simulink model "d2kontur_d2"  (R2014b)
settings: Solver=ode3  SolverMode=SingleTasking  StartTime=0.0  StopTime=10.0  RelTol=1e-3
PreLoadFcn:
  | waijung.modelPreload; % Required for working with Waijung Blockset. Do not remove.
undefined symbols (not defined in the file): FiO2, HCLK, HSEOSC, Link, LQFP100, ST, STM32F407VE
libraries: simulink_extras x8, stm32f4_io_lib x2, stm32f4_adc_lib x1, stm32f4_device_config_lib x1
(part 1 of 2)
CloseFcn:
  | waijung.modelClose; % Required for working with Waijung Blockset. Do not remove.
settings Model: Creator=Алексей  LastModifiedBy=Alex
settings OptimizationCC: OptimizeModelRefInitCode=on  LifeSpan=1
settings HardwareCC: ProdEndianess=LittleEndian  ProdHWDeviceType=ARM Compatible->Cortex - M4  TargetEndianess=LittleEndian  TargetHWDeviceType=ARM Compatible->Cortex - M4
settings RTWCC: SystemTargetFile=stm32f4.tlc  GenerateMakefile=off  TemplateMakefile=ert_default_tmf  Description=STM32F4 Target  ProcessScript=stm32f4_make_rtw_hook
settings CodeAppCC: IgnoreCustomStorageClasses=off
settings STFCustomTargetCC: ModelReferenceCompliant=off  CombineOutputUpdateFcns=on  ERTCustomFileBanners=on  SupportContinuousTime=off  SupportNonInlinedSFcns=off  MATLABClassNameForMDSCustomization=Simulink.SoftwareTarget.ERTCustomization  GRTInterface=off  SystemTargetFile=stm32f4.tlc
settings ERTTargetCC: ModelReferenceCompliant=off  ParMdlRefBuildCompliant=off  CompOptLevelCompliant=off  ConcurrentExecutionCompliant=off  ERTFirstTimeCompliant=off  ModelStepFunctionPrototypeControlCompliant=off  CPPClassGenCompliant=off  InlinedParameterPlacement=NonHierarchical  ERTSrcFileBannerTemplate=stm32f4_code_template.cgt  ERTHdrFileBannerTemplate=stm32f4_code_template.cgt  ERTDataSrcFileTemplate=stm32f4_code_template.cgt  ERTDataHdrFileTemplate=stm32f4_code_template.cgt  ERTCustomFileTemplate=stm32f4_file_process.tlc

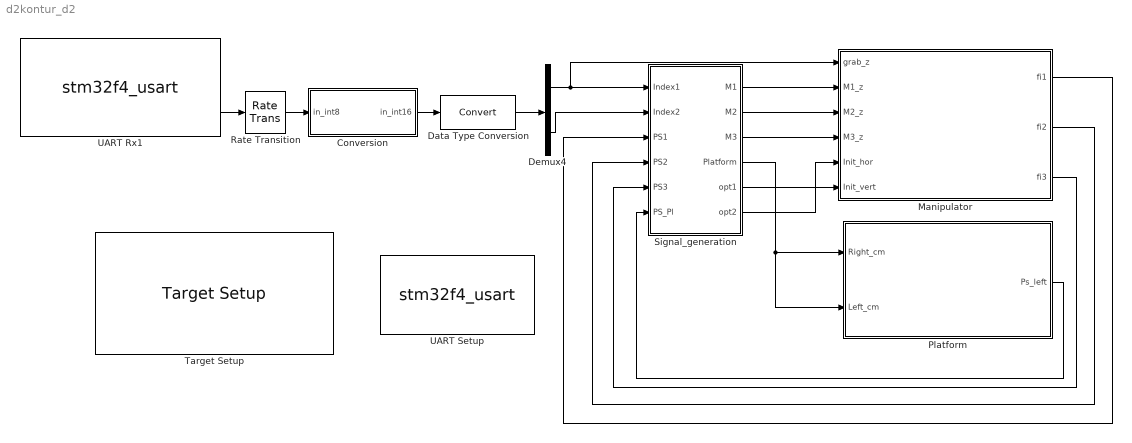
== system d2kontur_d2 ==
  Conversion : Subsystem
  Data Type Conversion : DataTypeConversion
  Demux4 : Demux  Outputs=2
  Manipulator : Subsystem
      mask Display:
      | port_label('input',1,'grab')
      | port_label('input',2,'M1')
      | port_label('input',3,'M2')
      | port_label('input',4,'M3')
      | port_label('input',5,'Init_h')
      | port_label('input',6,'Init_v')
      | port_label('output',1,'fi1')
      | port_label('output',2,'fi2')
      | port_label('output',3,'fi3')
  Platform : Subsystem
  Rate Transition : RateTransition  OutPortSampleTime=0.001
  Signal_generation : Subsystem
  Target Setup : stm32f4_device_config_lib/Target Setup  Priority=100  compiler=GNU ARM  previous_compiler=GNU ARM  mcu=STM32F407VE (LQFP100)  mcustr=STM32F407VE  clockconfig=FiO2 (HSEOSC-8MHz/HCLK-168MHz)  system_stm32f4xx_c_path=C:\waijung15_04a\targets\stm32f4_target\stm32f4\utils\STM32F4xx_AN3988_V1.0.1\stm32f4_default\hseosc8mhz  showmemoryconfiguration=off  stacksize=0x2000  heapsize=0x2000  enableautocompiledownload=on  fullchiperase=off  programmerinterface=ST-Link  editctrlstr=on  compilercontrolstr=$(patsubst %, -I%, .) -mcpu=cortex-m4 -mthumb -mthumb-interwork -mfloat-abi=hard -mfpu=fpv4-sp-d16 -ffast-math -Wall -Wextra -Ofast  assemblercontrolstr=$(patsubst %, -I%, .) -mcpu=cortex-m4 -mthumb -mthumb-interwork -mfloat-abi=hard -mfpu=fpv4-sp-d16 -ffast-math -Wall -Wextra -Ofast -Wa,-amhls=$(<:.s=.lst) -D__STACK_SIZE=$(STACK_SIZE) -D__HEAP_SIZE=$(HEAP_SIZE)  linkercontrolstr=-T$(LD_SCRIPT) -g -Wl,-Map=$(MAP),--cref,--no-warn-mismatch -mcpu=cortex-m4 -mthumb -mthumb-interwork -mfloat-abi=hard -mfpu=fpv4-sp-d16  runafterdownload=on  execprofile=None  profileruart=3  profilerbaud=500000  profilertxpin=D8  profilerinitstr=0.001,168000000,168000,500000,0  manualsetsampletime=on  sampletime=0.001  blockid=TargetSetup  systickreloadvalue=168000  hseval=8000000  lastprofileruart=3  hclk=168000000  flashorigin=0x8000000  flashlength=512k  ramorigin=0x20000000  ramlength=112k  useextram=off
  UART Rx1 : S-Function  Priority=1  FunctionName=stm32f4_usart  Parameters=configuration,uartmodule,transfer,baudrate,inputtype,outputtype,confstr,binheaderarray,binterminatorarray,asciiheader,asciiterminator,bindatalength,packetmode,varname,sampletime,sampletimestr,blockid  EnableBusSupport=off  mask(stm32f4_usart){configuration=Rx, uartmodule=3, baudrate=115200, databits=8, parity=No, stopbit=1, remaptxpin=Not used, remaprxpin=Not used, flowcontrol=None, remapctspin=Not used, remaprtspin=Not used, advanceoptions=off, rxbuffersize=512, txbuffersize=512, transfer=Non-Blocking, packetmode=Binary Vector, binheader='', binterminator='', porttype_double=0, porttype_single=0, porttype_int8=5, porttype_uint8=0, porttype_int16=0, porttype_uint16=0, porttype_int32=0, porttype_uint32=0, asciiformat='value=%d,%f', rx_asciiterminator=CRLF (0x0D 0x0A - "\r\n"), tx_asciiterminator=LF (0x0A - "\n"), storagename=<empty>, varname=, inputtype=[0], outputtype=[2 3  1282], binheaderarray=[0 ], binterminatorarray=[0 ], bindatalength=5, asciiheader='value=%d,%f\r\n', asciiterminator=[2 13 10], sampletime=0.01, sampletimestr=-1, blockid=UARTRx1, confstr=[ "dummy", "0", "*", "*", "0", "*", "*", "0", "*", "*", "0", "*", "*", "1", "4", "3", "1", "4", "1", "512", "512", "1", "3", "115200", "8", "No", "1", "None", "USART3"], lastmodule=1}
      mask prompts: uartmodule "UART Module"; baudrate "Baud rate (bps)"; databits "Data bits"; stopbit "Stop bit"; remaptxpin "Tx Pin"; remaprxpin "Rx Pin"; flowcontrol "Hardware flow control"; remapctspin "HW Flow control, CTS Pin"; remaprtspin "HW Flow control, RTS Pin"; advanceoptions "Advance options"; rxbuffersize "Rx buffer size (bytes)"; txbuffersize "Tx buffer size (bytes)"; packetmode "Packet mode"; binheader "Binary header (example: '7E 7E')"; binterminator "Binary terminator (example: '03 03')"; porttype_double "Number of data port, type DOUBLE"; porttype_single "Number of data port, type SINGLE"; porttype_int8 "Number of data port, type INT8"; porttype_uint8 "Number of data port, type UINT8"; porttype_int16 "Number of data port, type INT16"; porttype_uint16 "Number of data port, type UINT16"; porttype_int32 "Number of data port, type INT32"; porttype_uint32 "Number of data port, type UINT32"; asciiformat "Ascii format"; rx_asciiterminator "End of packet"; tx_asciiterminator "End of packet"; storagename "Buffer"; varname "Var name"; inputtype "Input data type"; outputtype "Output data type"; binheaderarray "Binary header"; binterminatorarray "Binary terminator"; bindatalength "Binary data length"; asciiheader "Ascii header (printf format)"; asciiterminator "Ascii terminator"; sampletime "Sample time (sec)"; sampletimestr "Compiled sample time (sec) in string"; confstr "Configuration string"; lastmodule "Last module selected"
      mask help:
      | Data type for Ascii format
      | %u, %i, %d, %o, %x: uint32
      | %e, %g, %f: single
      | %c: int8
      mask init:
      | stm32f4_usart_callback('init');
      mask Help: web(fullfile(waijungdocroot,'stm32f4_usart_rx.htm'), '-browser')
      mask TypeOptions configuration: Setup | Tx | Rx
      mask Callback configuration: stm32f4_usart_callback('configuration');
      mask TypeOptions uartmodule: 1 | 2 | 3 | 4 | 5 | 6
      mask Callback uartmodule: stm32f4_usart_callback('uartmodule');
      mask Callback baudrate: stm32f4_usart_callback('baudrate');
      mask TypeOptions databits: 8
      mask TypeOptions parity: No | Odd | Even
      mask TypeOptions stopbit: 0.5 | 1 | 1.5 | 2
      mask TypeOptions remaptxpin: Not used | A9 | B6
      mask TypeOptions remaprxpin: Not used | A10 | B7
      mask TypeOptions flowcontrol: None | RTS | CTS | RTS/CTS
      mask Callback flowcontrol: stm32f4_usart_callback('flowcontrol');
      mask TypeOptions remapctspin: Not used | A11
      mask TypeOptions remaprtspin: Not used | A12
      mask Callback advanceoptions: stm32f4_usart_callback('advanceoptions');
      mask TypeOptions rxbuffersize: 16 | 32 | 64 | 128 | 256 | 512 | 1024 | 2048
      mask TypeOptions txbuffersize: 16 | 32 | 64 | 128 | 256 | 512 | 1024 | 2048
      mask TypeOptions transfer: Blocking | Non-Blocking
      mask Callback transfer: stm32f4_usart_callback('transfer');
      mask TypeOptions packetmode: Ascii | Binary | Binary Vector | String Buffer | Raw Buffer
      mask Callback packetmode: stm32f4_usart_callback('packetmode');
      mask Callback binheader: stm32f4_usart_callback('binheader');
      mask Callback binterminator: stm32f4_usart_callback('binterminator');
      mask Callback porttype_double: stm32f4_usart_callback('porttype');
      mask Callback porttype_single: stm32f4_usart_callback('porttype');
      mask Callback porttype_int8: stm32f4_usart_callback('porttype');
      mask Callback porttype_uint8: stm32f4_usart_callback('porttype');
      mask Callback porttype_int16: stm32f4_usart_callback('porttype');
      mask Callback porttype_uint16: stm32f4_usart_callback('porttype');
      mask Callback porttype_int32: stm32f4_usart_callback('porttype');
      mask Callback porttype_uint32: stm32f4_usart_callback('porttype');
      mask Callback asciiformat: stm32f4_usart_callback('asciiformat');
      mask TypeOptions rx_asciiterminator: CR (0x0D - "\r") | LF (0x0A - "\n") | CRLF (0x0D 0x0A - "\r\n")
      mask Callback rx_asciiterminator: stm32f4_usart_callback('rx_asciiterminator');
      mask TypeOptions tx_asciiterminator: CR (0x0D - "\r") | LF (0x0A - "\n") | CRLF (0x0D 0x0A - "\r\n") | None
      mask Callback tx_asciiterminator: stm32f4_usart_callback('tx_asciiterminator');
      mask TypeOptions storagename: <empty>
      mask Callback storagename: stm32f4_usart_callback('storagename');
      mask Callback varname: stm32f4_usart_callback('varname');
      mask Callback sampletime: stm32f4_usart_callback('sampletime');
      mask Callback sampletimestr: stm32f4_usart_callback('sampletimestr');
      mask Callback blockid: stm32f4_usart_callback('blockid');
      mask Display: text(0.05, 0.5, 'Module: USART3_Rx\nPacket: Binary Vector\nTransfer: Non-Blocking\nTs (sec): -1','ver','middle','hor','left'); port_label('output', 1,'READY'); port_label('output', 2,'int8(5)');
  UART Setup : S-Function  Priority=1  FunctionName=stm32f4_usart  Parameters=configuration,uartmodule,transfer,baudrate,inputtype,outputtype,confstr,binheaderarray,binterminatorarray,asciiheader,asciiterminator,bindatalength,packetmode,varname,sampletime,sampletimestr,blockid  EnableBusSupport=off  mask(stm32f4_usart){configuration=Setup, uartmodule=3, baudrate=9600, databits=8, parity=No, stopbit=1, remaptxpin=D8, remaprxpin=D9, flowcontrol=None, remapctspin=Not used, remaprtspin=Not used, advanceoptions=off, rxbuffersize=512, txbuffersize=512, transfer=Blocking, packetmode=Ascii, binheader='7E 7E', binterminator='03 03', porttype_double=1, porttype_single=0, porttype_int8=1, porttype_uint8=0, porttype_int16=0, porttype_uint16=0, porttype_int32=0, porttype_uint32=0, asciiformat='%d,%f', rx_asciiterminator=CRLF (0x0D 0x0A - "\r\n"), tx_asciiterminator=CR (0x0D - "\r"), storagename=<empty>, varname=, inputtype=[0], outputtype=[0], binheaderarray=[0], binterminatorarray=[0], bindatalength=0, asciiheader='', asciiterminator=[0], sampletime=-1, sampletimestr=-1, blockid=UARTSetup, confstr=[ "dummy", "1", "D", "8", "1", "D", "9", "0", "*", "*", "0", "*", "*", "1", "4", "3", "1", "4", "1", "512", "512", "1", "3", "9600", "8", "No", "1", "None", "USART3"], lastmodule=3}
      mask prompts: uartmodule "UART Module"; baudrate "Baud rate (bps)"; databits "Data bits"; stopbit "Stop bit"; remaptxpin "Tx Pin"; remaprxpin "Rx Pin"; flowcontrol "Hardware flow control"; remapctspin "HW Flow control, CTS Pin"; remaprtspin "HW Flow control, RTS Pin"; advanceoptions "Advance options"; rxbuffersize "Rx buffer size (bytes)"; txbuffersize "Tx buffer size (bytes)"; packetmode "Packet mode"; binheader "Binary header (example: '7E 7E')"; binterminator "Binary terminator (example: '03 03')"; porttype_double "Number of data port, type DOUBLE"; porttype_single "Number of data port, type SINGLE"; porttype_int8 "Number of data port, type INT8"; porttype_uint8 "Number of data port, type UINT8"; porttype_int16 "Number of data port, type INT16"; porttype_uint16 "Number of data port, type UINT16"; porttype_int32 "Number of data port, type INT32"; porttype_uint32 "Number of data port, type UINT32"; asciiformat "Ascii format"; rx_asciiterminator "End of packet"; tx_asciiterminator "End of packet"; storagename "Buffer"; varname "Var name"; inputtype "Input data type"; outputtype "Output data type"; binheaderarray "Binary header"; binterminatorarray "Binary terminator"; bindatalength "Binary data length"; asciiheader "Ascii header (printf format)"; asciiterminator "Ascii terminator"; sampletime "Sample time (sec)"; sampletimestr "Compiled sample time (sec) in string"; confstr "Configuration string"; lastmodule "Last module selected"
      mask help:
      | Default STM32F4DISCOVERY + aMG F4 Connect 2 + aMG USB Converter N2 settings use
      |
      | USART3, Tx D8, Rx D9 and USB Serial Converter A.
      mask init:
      | stm32f4_usart_callback('init');
      mask Help: web(fullfile(waijungdocroot,'stm32f4_usart_setup.htm'), '-browser')
      mask TypeOptions configuration: Setup | Tx | Rx
      mask Callback configuration: stm32f4_usart_callback('configuration');
      mask TypeOptions uartmodule: 1 | 2 | 3 | 4 | 5 | 6
      mask Callback uartmodule: stm32f4_usart_callback('uartmodule');
      mask Callback baudrate: stm32f4_usart_callback('baudrate');
      mask TypeOptions databits: 8
      mask TypeOptions parity: No | Odd | Even
      mask TypeOptions stopbit: 0.5 | 1 | 1.5 | 2
      mask TypeOptions remaptxpin: Not used | B10 | C10 | D8
      mask TypeOptions remaprxpin: Not used | B11 | C11 | D9
      mask TypeOptions flowcontrol: None | RTS | CTS | RTS/CTS
      mask Callback flowcontrol: stm32f4_usart_callback('flowcontrol');
      mask TypeOptions remapctspin: Not used | B13 | D11
      mask TypeOptions remaprtspin: Not used | B14 | D12
      mask Callback advanceoptions: stm32f4_usart_callback('advanceoptions');
      mask TypeOptions rxbuffersize: 16 | 32 | 64 | 128 | 256 | 512 | 1024 | 2048
      mask TypeOptions txbuffersize: 16 | 32 | 64 | 128 | 256 | 512 | 1024 | 2048
      mask TypeOptions transfer: Blocking | Non-Blocking
      mask Callback transfer: stm32f4_usart_callback('transfer');
      mask TypeOptions packetmode: Ascii | Binary | String Buffer
      mask Callback packetmode: stm32f4_usart_callback('packetmode');
      mask Callback binheader: stm32f4_usart_callback('binheader');
      mask Callback binterminator: stm32f4_usart_callback('binterminator');
      mask Callback porttype_double: stm32f4_usart_callback('porttype');
      mask Callback porttype_single: stm32f4_usart_callback('porttype');
      mask Callback porttype_int8: stm32f4_usart_callback('porttype');
      mask Callback porttype_uint8: stm32f4_usart_callback('porttype');
      mask Callback porttype_int16: stm32f4_usart_callback('porttype');
      mask Callback porttype_uint16: stm32f4_usart_callback('porttype');
      mask Callback porttype_int32: stm32f4_usart_callback('porttype');
      mask Callback porttype_uint32: stm32f4_usart_callback('porttype');
      mask Callback asciiformat: stm32f4_usart_callback('asciiformat');
      mask TypeOptions rx_asciiterminator: CR (0x0D - "\r") | LF (0x0A - "\n") | CRLF (0x0D 0x0A - "\r\n")
      mask Callback rx_asciiterminator: stm32f4_usart_callback('rx_asciiterminator');
      mask TypeOptions tx_asciiterminator: CR (0x0D - "\r") | LF (0x0A - "\n") | CRLF (0x0D 0x0A - "\r\n") | None
      mask Callback tx_asciiterminator: stm32f4_usart_callback('tx_asciiterminator');
      mask TypeOptions storagename: <empty>
      mask Callback storagename: stm32f4_usart_callback('storagename');
      mask Callback varname: stm32f4_usart_callback('varname');
      mask Callback sampletime: stm32f4_usart_callback('sampletime');
      mask Callback sampletimestr: stm32f4_usart_callback('sampletimestr');
      mask Callback blockid: stm32f4_usart_callback('blockid');
      mask Display: text(0.5, 0.5, 'Module: USART3_Setup\nBaud (Bps): 9600\nDMA Buffer: 512/512\nTx/Rx Pin: D8/D9','ver','middle','hor','center');
  wires:
  UART Rx1/2 -> Rate Transition/1
  Rate Transition/1 -> Conversion/1(in_int8)
  Data Type Conversion/1 -> Demux4/1
  Demux4/1 -> Manipulator/1(grab_z), Signal_generation/1(Index1)
  Demux4/2 -> Signal_generation/2(Index2)
  Signal_generation/4(Platform) -> Platform/2(Left_cm), Platform/1(Right_cm)
  Platform/1(Ps_left) -> Signal_generation/6(PS_Pl)
  Signal_generation/1(M1) -> Manipulator/2(M1_z)
  Signal_generation/2(M2) -> Manipulator/3(M2_z)
  Signal_generation/3(M3) -> Manipulator/4(M3_z)
  Signal_generation/5(opt1) -> Manipulator/5(Init_hor)
  Signal_generation/6(opt2) -> Manipulator/6(Init_vert)
  Manipulator/1(fi1) -> Signal_generation/3(PS1)
  Manipulator/2(fi2) -> Signal_generation/4(PS2)
  Manipulator/3(fi3) -> Signal_generation/5(PS3)
  Conversion/1(in_int16) -> Data Type Conversion/1

== system d2kontur_d2/Conversion ==
  in_int8 : Inport
  Data Type Conversion : DataTypeConversion  OutDataTypeStr=int16
  Data Type Conversion2 : DataTypeConversion  OutDataTypeStr=int16
  Demux : Demux  Outputs=5
  Mux : Mux  Inputs=2
  Product : Product
  Sum : Sum  Inputs=+++
  in_int16 : Outport
  wires:
  in_int8/1 -> Data Type Conversion/1
  Demux/1 -> Sum/1
  Demux/2 -> Sum/2
  Demux/3 -> Sum/3
  Sum/1 -> Product/1
  Demux/4 -> Product/2
  Product/1 -> Data Type Conversion2/1
  Demux/5 -> Mux/2
  Data Type Conversion/1 -> Demux/1
  Mux/1 -> in_int16/1
  Data Type Conversion2/1 -> Mux/1

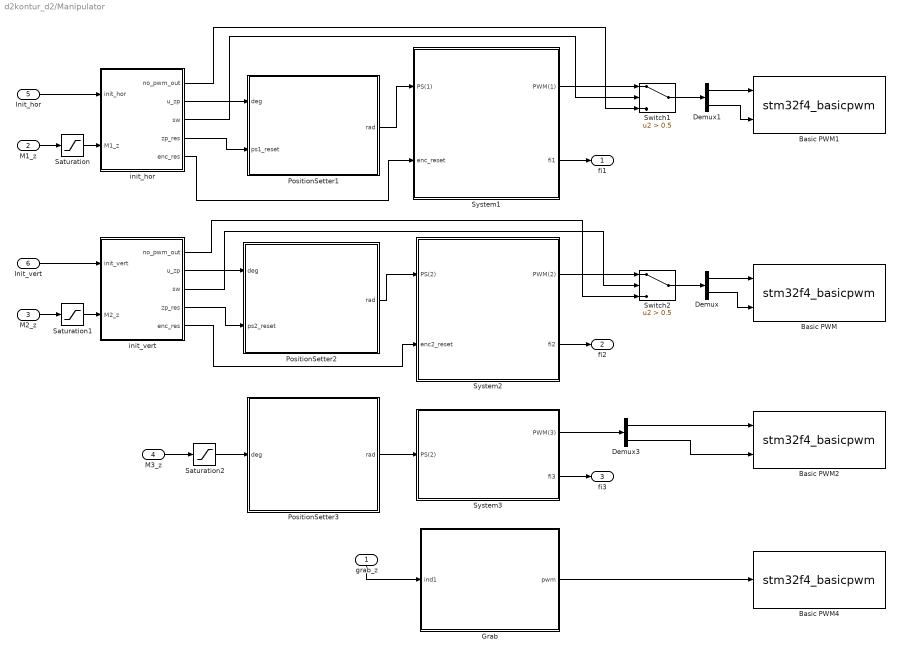
== system d2kontur_d2/Manipulator ==
  grab_z : Inport
  M1_z : Inport  Port=2
  M2_z : Inport  Port=3
  M3_z : Inport  Port=4
  Init_hor : Inport  Port=5
  Init_vert : Inport  Port=6
  Basic PWM : S-Function  FunctionName=stm32f4_basicpwm  Parameters=timer,pwmperiod,ch1pin,ch2pin,ch3pin,ch4pin,sampletime,sampletimestr,blockid,apb,portstr,pinstr,pinmat,timarr,timprescale,chmat,polaritystr  EnableBusSupport=off  mask(stm32f4_basicpwm){timer=9, pwmperiod=0.0001, polarity=Active High, polaritystr=TIM_OCPolarity_High, ch1pin=E5, ch2pin=E6, ch3pin=Not available - Do not use, ch4pin=Not available - Do not use, sampletime=0.001, sampletimestr=-1, blockid=ManipulatorBasicPWM, portpinstr=E5,E6,,, enablecustomportlabel=off, cinputportlabel=In1, In2, In3, In4, coutputportlabel=0, apb=2, portstr=["E"], pinstr=["GPIO_Pin_5 | GPIO_Pin_6"], pinmat=[2 5 6], timarr=16799, timprescale=0, chmat=[1  2]}
      mask prompts: pwmperiod "PWM Period (seconds)"; ch1pin "Channel 1"; ch2pin "Channel 2"; ch3pin "Channel 3"; ch4pin "Channel 4"; sampletime "Sample time (sec)"; sampletimestr "Compiled sample time (sec) in string"; portpinstr "Port pin string"; enablecustomportlabel "Enable custom port labels"; cinputportlabel "Custom input port labels (Ex. In1, In2, In3)"; coutputportlabel "Custom output port labels (Ex. Out1, Out2, Out3)"; portstr "Port string"; pinstr "Pin string"; pinmat "Pin matrix"; timarr "Timer ARR"; timprescale "Timer PRESCALE"; chmat "Channel order"
      mask help:
      | This block implements basic Edge-aligned Pulse Width Modulation (PWM) generation.
      | All timers are 16-bit. The PWM period is fixed (per timer).
      mask init:
      | stm32f4_basicpwm_callback('init');
      mask Help: web(fullfile(waijungdocroot,'stm32f4_basicpwm.htm'),'-browser')
      mask TypeOptions timer: 1 | 2 | 3 | 4 | 5 | 8 | 9 | 10 | 11 | 12 | 13 | 14
      mask Callback timer: stm32f4_basicpwm_callback('timer');
      mask Callback pwmperiod: stm32f4_basicpwm_callback('pwmperiod');
      mask TypeOptions polarity: Active High | Active Low
      mask Callback polarity: stm32f4_basicpwm_callback('polarity');
      mask TypeOptions ch1pin: Not available - Do not use | A2 | E5
      mask Callback ch1pin: stm32f4_basicpwm_callback('ch1pin');
      mask TypeOptions ch2pin: Not available - Do not use | A3 | E6
      mask Callback ch2pin: stm32f4_basicpwm_callback('ch2pin');
      mask TypeOptions ch3pin: Not available - Do not use
      mask Callback ch3pin: stm32f4_basicpwm_callback('ch3pin');
      mask TypeOptions ch4pin: Not available - Do not use
      mask Callback ch4pin: stm32f4_basicpwm_callback('ch4pin');
      mask Callback sampletime: stm32f4_basicpwm_callback('sampletime');
      mask Callback sampletimestr: stm32f4_basicpwm_callback('sampletimestr');
      mask Callback blockid: stm32f4_basicpwm_callback('blockid');
      mask Callback enablecustomportlabel: stm32f4_basicpwm_callback('enablecustomportlabel');
      mask Display: text(0.95, 0.5, 'Timer: 9\nPolarity: Active High\nPeriod (sec) 0.0001\nTs (sec): -1','ver','middle','hor','right');port_label('input', 1,'CH1 (E5)');port_label('input', 2,'CH2 (E6)')
  Basic PWM1 : S-Function  FunctionName=stm32f4_basicpwm  Parameters=timer,pwmperiod,ch1pin,ch2pin,ch3pin,ch4pin,sampletime,sampletimestr,blockid,apb,portstr,pinstr,pinmat,timarr,timprescale,chmat,polaritystr  EnableBusSupport=off  mask(stm32f4_basicpwm){timer=5, pwmperiod=0.0001, polarity=Active High, polaritystr=TIM_OCPolarity_High, ch1pin=Not available - Do not use, ch2pin=Not available - Do not use, ch3pin=A2, ch4pin=A3, sampletime=0.001, sampletimestr=-1, blockid=ManipulatorBasicPWM1, portpinstr=,,A2,A3, enablecustomportlabel=off, cinputportlabel=In1, In2, In3, In4, coutputportlabel=0, apb=1, portstr=["A"], pinstr=["GPIO_Pin_2 | GPIO_Pin_3"], pinmat=[2 2 3], timarr=8399, timprescale=0, chmat=[3  4]}
      mask prompts: pwmperiod "PWM Period (seconds)"; ch1pin "Channel 1"; ch2pin "Channel 2"; ch3pin "Channel 3"; ch4pin "Channel 4"; sampletime "Sample time (sec)"; sampletimestr "Compiled sample time (sec) in string"; portpinstr "Port pin string"; enablecustomportlabel "Enable custom port labels"; cinputportlabel "Custom input port labels (Ex. In1, In2, In3)"; coutputportlabel "Custom output port labels (Ex. Out1, Out2, Out3)"; portstr "Port string"; pinstr "Pin string"; pinmat "Pin matrix"; timarr "Timer ARR"; timprescale "Timer PRESCALE"; chmat "Channel order"
      mask help:
      | This block implements basic Edge-aligned Pulse Width Modulation (PWM) generation.
      | All timers are 16-bit. The PWM period is fixed (per timer).
      mask init:
      | stm32f4_basicpwm_callback('init');
      mask Help: web(fullfile(waijungdocroot,'stm32f4_basicpwm.htm'),'-browser')
      mask TypeOptions timer: 1 | 2 | 3 | 4 | 5 | 8 | 9 | 10 | 11 | 12 | 13 | 14
      mask Callback timer: stm32f4_basicpwm_callback('timer');
      mask Callback pwmperiod: stm32f4_basicpwm_callback('pwmperiod');
      mask TypeOptions polarity: Active High | Active Low
      mask Callback polarity: stm32f4_basicpwm_callback('polarity');
      mask TypeOptions ch1pin: Not available - Do not use | A0 | A5
      mask Callback ch1pin: stm32f4_basicpwm_callback('ch1pin');
      mask TypeOptions ch2pin: Not available - Do not use | A1 | B3
      mask Callback ch2pin: stm32f4_basicpwm_callback('ch2pin');
      mask TypeOptions ch3pin: Not available - Do not use | A2 | B10
      mask Callback ch3pin: stm32f4_basicpwm_callback('ch3pin');
      mask TypeOptions ch4pin: Not available - Do not use | A3 | B11
      mask Callback ch4pin: stm32f4_basicpwm_callback('ch4pin');
      mask Callback sampletime: stm32f4_basicpwm_callback('sampletime');
      mask Callback sampletimestr: stm32f4_basicpwm_callback('sampletimestr');
      mask Callback blockid: stm32f4_basicpwm_callback('blockid');
      mask Callback enablecustomportlabel: stm32f4_basicpwm_callback('enablecustomportlabel');
      mask Display: text(0.95, 0.5, 'Timer: 5\nPolarity: Active High\nPeriod (sec) 0.0001\nTs (sec): -1','ver','middle','hor','right');port_label('input', 1,'CH3 (A2)');port_label('input', 2,'CH4 (A3)')
  Basic PWM2 : S-Function  FunctionName=stm32f4_basicpwm  Parameters=timer,pwmperiod,ch1pin,ch2pin,ch3pin,ch4pin,sampletime,sampletimestr,blockid,apb,portstr,pinstr,pinmat,timarr,timprescale,chmat,polaritystr  EnableBusSupport=off  mask(stm32f4_basicpwm){timer=12, pwmperiod=0.0001, polarity=Active High, polaritystr=TIM_OCPolarity_High, ch1pin=B14, ch2pin=B15, ch3pin=Not available - Do not use, ch4pin=Not available - Do not use, sampletime=0.001, sampletimestr=-1, blockid=ManipulatorBasicPWM2, portpinstr=B14,B15,,, enablecustomportlabel=off, cinputportlabel=In1, In2, In3, In4, coutputportlabel=0, apb=1, portstr=["B"], pinstr=["GPIO_Pin_14 | GPIO_Pin_15"], pinmat=[2 14 15], timarr=8399, timprescale=0, chmat=[1  2]}
      mask prompts: pwmperiod "PWM Period (seconds)"; ch1pin "Channel 1"; ch2pin "Channel 2"; ch3pin "Channel 3"; ch4pin "Channel 4"; sampletime "Sample time (sec)"; sampletimestr "Compiled sample time (sec) in string"; portpinstr "Port pin string"; enablecustomportlabel "Enable custom port labels"; cinputportlabel "Custom input port labels (Ex. In1, In2, In3)"; coutputportlabel "Custom output port labels (Ex. Out1, Out2, Out3)"; portstr "Port string"; pinstr "Pin string"; pinmat "Pin matrix"; timarr "Timer ARR"; timprescale "Timer PRESCALE"; chmat "Channel order"
      mask help:
      | This block implements basic Edge-aligned Pulse Width Modulation (PWM) generation.
      | All timers are 16-bit. The PWM period is fixed (per timer).
      mask init:
      | stm32f4_basicpwm_callback('init');
      mask Help: web(fullfile(waijungdocroot,'stm32f4_basicpwm.htm'),'-browser')
      mask TypeOptions timer: 1 | 2 | 3 | 4 | 5 | 8 | 9 | 10 | 11 | 12 | 13 | 14
      mask Callback timer: stm32f4_basicpwm_callback('timer');
      mask Callback pwmperiod: stm32f4_basicpwm_callback('pwmperiod');
      mask TypeOptions polarity: Active High | Active Low
      mask Callback polarity: stm32f4_basicpwm_callback('polarity');
      mask TypeOptions ch1pin: Not available - Do not use | B14
      mask Callback ch1pin: stm32f4_basicpwm_callback('ch1pin');
      mask TypeOptions ch2pin: Not available - Do not use | B15
      mask Callback ch2pin: stm32f4_basicpwm_callback('ch2pin');
      mask TypeOptions ch3pin: Not available - Do not use
      mask Callback ch3pin: stm32f4_basicpwm_callback('ch3pin');
      mask TypeOptions ch4pin: Not available - Do not use
      mask Callback ch4pin: stm32f4_basicpwm_callback('ch4pin');
      mask Callback sampletime: stm32f4_basicpwm_callback('sampletime');
      mask Callback sampletimestr: stm32f4_basicpwm_callback('sampletimestr');
      mask Callback blockid: stm32f4_basicpwm_callback('blockid');
      mask Callback enablecustomportlabel: stm32f4_basicpwm_callback('enablecustomportlabel');
      mask Display: text(0.95, 0.5, 'Timer: 12\nPolarity: Active High\nPeriod (sec) 0.0001\nTs (sec): -1','ver','middle','hor','right');port_label('input', 1,'CH1 (B14)');port_label('input', 2,'CH2 (B15)')
  Basic PWM4 : S-Function  FunctionName=stm32f4_basicpwm  Parameters=timer,pwmperiod,ch1pin,ch2pin,ch3pin,ch4pin,sampletime,sampletimestr,blockid,apb,portstr,pinstr,pinmat,timarr,timprescale,chmat,polaritystr  EnableBusSupport=off  mask(stm32f4_basicpwm){timer=14, pwmperiod=0.02, polarity=Active High, polaritystr=TIM_OCPolarity_High, ch1pin=A7, ch2pin=Not available - Do not use, ch3pin=Not available - Do not use, ch4pin=Not available - Do not use, sampletime=0.001, sampletimestr=-1, blockid=ManipulatorBasicPWM4, portpinstr=A7,,,, enablecustomportlabel=off, cinputportlabel=In1, In2, In3, In4, coutputportlabel=0, apb=1, portstr=["A"], pinstr=["GPIO_Pin_7"], pinmat=[1 7], timarr=59999, timprescale=27, chmat=[1]}
      mask prompts: pwmperiod "PWM Period (seconds)"; ch1pin "Channel 1"; ch2pin "Channel 2"; ch3pin "Channel 3"; ch4pin "Channel 4"; sampletime "Sample time (sec)"; sampletimestr "Compiled sample time (sec) in string"; portpinstr "Port pin string"; enablecustomportlabel "Enable custom port labels"; cinputportlabel "Custom input port labels (Ex. In1, In2, In3)"; coutputportlabel "Custom output port labels (Ex. Out1, Out2, Out3)"; portstr "Port string"; pinstr "Pin string"; pinmat "Pin matrix"; timarr "Timer ARR"; timprescale "Timer PRESCALE"; chmat "Channel order"
      mask help:
      | This block implements basic Edge-aligned Pulse Width Modulation (PWM) generation.
      | All timers are 16-bit. The PWM period is fixed (per timer).
      mask init:
      | stm32f4_basicpwm_callback('init');
      mask Help: web(fullfile(waijungdocroot,'stm32f4_basicpwm.htm'),'-browser')
      mask TypeOptions timer: 1 | 2 | 3 | 4 | 5 | 8 | 9 | 10 | 11 | 12 | 13 | 14
      mask Callback timer: stm32f4_basicpwm_callback('timer');
      mask Callback pwmperiod: stm32f4_basicpwm_callback('pwmperiod');
      mask TypeOptions polarity: Active High | Active Low
      mask Callback polarity: stm32f4_basicpwm_callback('polarity');
      mask TypeOptions ch1pin: Not available - Do not use | A7
      mask Callback ch1pin: stm32f4_basicpwm_callback('ch1pin');
      mask TypeOptions ch2pin: Not available - Do not use
      mask Callback ch2pin: stm32f4_basicpwm_callback('ch2pin');
      mask TypeOptions ch3pin: Not available - Do not use
      mask Callback ch3pin: stm32f4_basicpwm_callback('ch3pin');
      mask TypeOptions ch4pin: Not available - Do not use
      mask Callback ch4pin: stm32f4_basicpwm_callback('ch4pin');
      mask Callback sampletime: stm32f4_basicpwm_callback('sampletime');
      mask Callback sampletimestr: stm32f4_basicpwm_callback('sampletimestr');
      mask Callback blockid: stm32f4_basicpwm_callback('blockid');
      mask Callback enablecustomportlabel: stm32f4_basicpwm_callback('enablecustomportlabel');
      mask Display: text(0.95, 0.5, 'Timer: 14\nPolarity: Active High\nPeriod (sec) 0.02\nTs (sec): -1','ver','middle','hor','right');port_label('input', 1,'CH1 (A7)')
  Demux : Demux  Outputs=2
  Demux1 : Demux  Outputs=2
  Demux3 : Demux  Outputs=2
  Grab : Subsystem
  "PositionSetter1 " : Subsystem
  PositionSetter2 : Subsystem
  PositionSetter3 : Subsystem
  Saturation : Saturate  UpperLimit=120  LowerLimit=-120
  Saturation1 : Saturate  UpperLimit=35  LowerLimit=-200
  Saturation2 : Saturate  UpperLimit=180  LowerLimit=-180
  Switch1 : Switch  Criteria=u2 > Threshold  Threshold=0.5
  Switch2 : Switch  Criteria=u2 > Threshold  Threshold=0.5
  System1 : Subsystem
  System2 : Subsystem
  System3 : Subsystem
  init_hor : Subsystem
  init_vert : Subsystem
  fi1 : Outport
  fi2 : Outport  Port=2
  fi3 : Outport  Port=3
  wires:
  Demux3/2 -> Basic PWM2/2
  Demux/2 -> Basic PWM/2
  Demux1/2 -> Basic PWM1/2
  Demux1/1 -> Basic PWM1/1
  System2/2(fi2) -> fi2/1
  PositionSetter3/1(rad) -> System3/1(PS(2))
  init_hor/3(sw) -> Switch1/2
  System1/2(fi1) -> fi1/1
  Switch1/1 -> Demux1/1
  Demux/1 -> Basic PWM/1
  M1_z/1 -> Saturation/1
  System3/1(PWM(3)) -> Demux3/1
  System3/2(fi3) -> fi3/1
  init_hor/1(no_pwm_out) -> Switch1/3
  Init_hor/1 -> init_hor/1(init_hor)
  System2/1(PWM(2)) -> Switch2/1
  init_vert/1(no_pwm_out) -> Switch2/3
  init_hor/5(enc_res) -> System1/2(enc_reset)
  init_vert/3(sw) -> Switch2/2
  M3_z/1 -> Saturation2/1
  System1/1(PWM(1)) -> Switch1/1
  init_vert/2(u_zp) -> PositionSetter2/1(deg)
  PositionSetter2/1(rad) -> System2/1(PS(2))
  init_hor/4(zp_res) -> "PositionSetter1 "/2(ps1_reset)
  "PositionSetter1 "/1("rad ") -> System1/1(PS(1))
  Switch2/1 -> Demux/1
  Grab/1(pwm) -> Basic PWM4/1
  init_hor/2(u_zp) -> "PositionSetter1 "/1("deg ")
  Demux3/1 -> Basic PWM2/1
  init_vert/4(zp_res) -> PositionSetter2/2(ps2_reset)
  M2_z/1 -> Saturation1/1
  Init_vert/1 -> init_vert/1(init_vert)
  Saturation/1 -> init_hor/2(M1_z)
  init_vert/5(enc_res) -> System2/2(enc2_reset)
  Saturation2/1 -> PositionSetter3/1(deg)
  Saturation1/1 -> init_vert/2(M2_z)
  grab_z/1 -> Grab/1(ind1)

== system d2kontur_d2/Platform ==
  Right_cm : Inport
  Left_cm : Inport  Port=2
  Basic PWM1 : S-Function  FunctionName=stm32f4_basicpwm  Parameters=timer,pwmperiod,ch1pin,ch2pin,ch3pin,ch4pin,sampletime,sampletimestr,blockid,apb,portstr,pinstr,pinmat,timarr,timprescale,chmat,polaritystr  EnableBusSupport=off  mask(stm32f4_basicpwm){timer=8, pwmperiod=0.0001, polarity=Active High, polaritystr=TIM_OCPolarity_High, ch1pin=C6, ch2pin=C7, ch3pin=C8, ch4pin=C9, sampletime=0.001, sampletimestr=-1, blockid=TankBasicPWM1, portpinstr=C6,C7,C8,C9, enablecustomportlabel=off, cinputportlabel=In1, In2, In3, In4, coutputportlabel=0, apb=2, portstr=["C"], pinstr=["GPIO_Pin_6 | GPIO_Pin_7 | GPIO_Pin_8 | GPIO_Pin_9"], pinmat=[4 6 7 8 9], timarr=16799, timprescale=0, chmat=[1  2  3  4]}
      mask prompts: pwmperiod "PWM Period (seconds)"; ch1pin "Channel 1"; ch2pin "Channel 2"; ch3pin "Channel 3"; ch4pin "Channel 4"; sampletime "Sample time (sec)"; sampletimestr "Compiled sample time (sec) in string"; portpinstr "Port pin string"; enablecustomportlabel "Enable custom port labels"; cinputportlabel "Custom input port labels (Ex. In1, In2, In3)"; coutputportlabel "Custom output port labels (Ex. Out1, Out2, Out3)"; portstr "Port string"; pinstr "Pin string"; pinmat "Pin matrix"; timarr "Timer ARR"; timprescale "Timer PRESCALE"; chmat "Channel order"
      mask help:
      | This block implements basic Edge-aligned Pulse Width Modulation (PWM) generation.
      | All timers are 16-bit. The PWM period is fixed (per timer).
      mask init:
      | stm32f4_basicpwm_callback('init');
      mask Help: web(fullfile(waijungdocroot,'stm32f4_basicpwm.htm'),'-browser')
      mask TypeOptions timer: 1 | 2 | 3 | 4 | 5 | 8 | 9 | 10 | 11 | 12 | 13 | 14
      mask Callback timer: stm32f4_basicpwm_callback('timer');
      mask Callback pwmperiod: stm32f4_basicpwm_callback('pwmperiod');
      mask TypeOptions polarity: Active High | Active Low
      mask Callback polarity: stm32f4_basicpwm_callback('polarity');
      mask TypeOptions ch1pin: Not available - Do not use | C6
      mask Callback ch1pin: stm32f4_basicpwm_callback('ch1pin');
      mask TypeOptions ch2pin: Not available - Do not use | C7
      mask Callback ch2pin: stm32f4_basicpwm_callback('ch2pin');
      mask TypeOptions ch3pin: Not available - Do not use | C8
      mask Callback ch3pin: stm32f4_basicpwm_callback('ch3pin');
      mask TypeOptions ch4pin: Not available - Do not use | C9
      mask Callback ch4pin: stm32f4_basicpwm_callback('ch4pin');
      mask Callback sampletime: stm32f4_basicpwm_callback('sampletime');
      mask Callback sampletimestr: stm32f4_basicpwm_callback('sampletimestr');
      mask Callback blockid: stm32f4_basicpwm_callback('blockid');
      mask Callback enablecustomportlabel: stm32f4_basicpwm_callback('enablecustomportlabel');
      mask Display: text(0.95, 0.5, 'Timer: 8\nPolarity: Active High\nPeriod (sec) 0.0001\nTs (sec): -1','ver','middle','hor','right');port_label('input', 1,'CH1 (C6)');port_label('input', 2,'CH2 (C7)');port_label('input', 3,'CH3 (C8)');port_label('input', 4,'CH4 (C9)')
  Encoder Read : S-Function  FunctionName=stm32f4_encoderread  Parameters=sampletime,sampletimestr,blockid,timer,apb,portstr,pinstr,pinmat,chmat,filterstr,filter,factor,rstcnt,ppr  EnableBusSupport=off  mask(stm32f4_encoderread){timer=1, ch1=A8, ch2=A9, ppr=15000, rstcnt=off, filterstr=No filter; sampling is done at fDTS, sampletime=0.001, sampletimestr=-1, blockid=TankEncoderRead, absresetinput=off, portpinstr=A8,A9, portstr=["A"], pinstr=["GPIO_Pin_8 | GPIO_Pin_9"], pinmat=[2 8 9], chmat=[1  2], apb=2, filter=0, factor=4}
      mask prompts: ch1 "Channel A Input Pin"; ch2 "Channel B Input Pin"; ppr "PPR (Number of pulses generated per revolution)"; rstcnt "Reset counter after every counter read"; filterstr "Built-in Input Capture Filter"; sampletime "Sample time (sec)"; sampletimestr "Compiled sample time (sec) in string"; absresetinput "Enable absolute position reset input signal"; portpinstr "Port pin string"; portstr "Port string"; pinstr "Pin string"; pinmat "Pin matrix"; chmat "Channel order"; filter "Filter ID"
      mask help:
      | The output Direction (uint32) is the direction of rotation either 0 or 1.
      |
      | The output Position (count) (uint32) is the count of number of edges of the encoder output signals from either channel A and B. The decoder is set to count at every rising and falling edge of both channel A and B (4x) or (x2) for one channel. For example, if an encoder has 180 pulses per revolution (PPS) and two channels are selected, the maximum count is 720 per revolution (4x180 = 720), i.e. from 0 to 719.
      mask init:
      | stm32f4_encoderread_callback('init');
      mask Help: web(fullfile(waijungdocroot,'stm32f4_encoderread.htm'),'-browser')
      mask TypeOptions timer: 1 | 2 | 3 | 4 | 5 | 8
      mask Callback timer: stm32f4_encoderread_callback('timer');
      mask TypeOptions ch1: Not available - Do not use | E9 | A8
      mask Callback ch1: stm32f4_encoderread_callback('chA');
      mask TypeOptions ch2: Not available - Do not use | E11 | A9
      mask Callback ch2: stm32f4_encoderread_callback('chB');
      mask Callback ppr: stm32f4_encoderread_callback('ppr');
      mask Callback rstcnt: stm32f4_encoderread_callback('rstcnt');
      mask TypeOptions filterstr: No filter; sampling is done at fDTS | fSAMPLING=fCK_INT; N=2 | fSAMPLING=fCK_INT; N=4 | fSAMPLING=fCK_INT; N=8 | fSAMPLING=fDTS/2; N=6 | fSAMPLING=fDTS/2; N=8 | fSAMPLING=fDTS/4; N=6 | fSAMPLING=fDTS/4; N=8 | fSAMPLING=fDTS/8; N=6 | fSAMPLING=fDTS/8; N=8 | fSAMPLING=fDTS/16; N=5 | fSAMPLING=fDTS/16; N=6 | fSAMPLING=fDTS/16; N=8 | fSAMPLING=fDTS/32; N=5 | fSAMPLING=fDTS/32; N=6 | fSAMPLING=fDTS/32; N=8
      mask Callback filterstr: stm32f4_encoderread_callback('filterstr');
      mask Callback sampletimestr: stm32f4_encoderread_callback('sampletimestr');
      mask Callback blockid: stm32f4_encoderread_callback('blockid');
      mask Display: text(0.05, 0.5, 'Timer: 1\nInput pins [CH_A, CH_B]: [A8,A9]\nRST Counter: No\nTs (sec): -1','ver','middle','hor','left');port_label('output', 1, 'Direction');port_label('output', 2, 'Position (count)')
  Encoder Read1 : S-Function  FunctionName=stm32f4_encoderread  Parameters=sampletime,sampletimestr,blockid,timer,apb,portstr,pinstr,pinmat,chmat,filterstr,filter,factor,rstcnt,ppr  EnableBusSupport=off  mask(stm32f4_encoderread){timer=2, ch1=A0, ch2=A1, ppr=15000, rstcnt=off, filterstr=No filter; sampling is done at fDTS, sampletime=0.001, sampletimestr=-1, blockid=TankEncoderRead1, absresetinput=off, portpinstr=A0,A1, portstr=["A"], pinstr=["GPIO_Pin_0 | GPIO_Pin_1"], pinmat=[2 0 1], chmat=[1  2], apb=1, filter=0, factor=4}
      mask prompts: ch1 "Channel A Input Pin"; ch2 "Channel B Input Pin"; ppr "PPR (Number of pulses generated per revolution)"; rstcnt "Reset counter after every counter read"; filterstr "Built-in Input Capture Filter"; sampletime "Sample time (sec)"; sampletimestr "Compiled sample time (sec) in string"; absresetinput "Enable absolute position reset input signal"; portpinstr "Port pin string"; portstr "Port string"; pinstr "Pin string"; pinmat "Pin matrix"; chmat "Channel order"; filter "Filter ID"
      mask help:
      | The output Direction (uint32) is the direction of rotation either 0 or 1.
      |
      | The output Position (count) (uint32) is the count of number of edges of the encoder output signals from either channel A and B. The decoder is set to count at every rising and falling edge of both channel A and B (4x) or (x2) for one channel. For example, if an encoder has 180 pulses per revolution (PPS) and two channels are selected, the maximum count is 720 per revolution (4x180 = 720), i.e. from 0 to 719.
      mask init:
      | stm32f4_encoderread_callback('init');
      mask Help: web(fullfile(waijungdocroot,'stm32f4_encoderread.htm'),'-browser')
      mask TypeOptions timer: 1 | 2 | 3 | 4 | 5 | 8
      mask Callback timer: stm32f4_encoderread_callback('timer');
      mask TypeOptions ch1: Not available - Do not use | A0 | A5
      mask Callback ch1: stm32f4_encoderread_callback('chA');
      mask TypeOptions ch2: Not available - Do not use | A1 | B3
      mask Callback ch2: stm32f4_encoderread_callback('chB');
      mask Callback ppr: stm32f4_encoderread_callback('ppr');
      mask Callback rstcnt: stm32f4_encoderread_callback('rstcnt');
      mask TypeOptions filterstr: No filter; sampling is done at fDTS | fSAMPLING=fCK_INT; N=2 | fSAMPLING=fCK_INT; N=4 | fSAMPLING=fCK_INT; N=8 | fSAMPLING=fDTS/2; N=6 | fSAMPLING=fDTS/2; N=8 | fSAMPLING=fDTS/4; N=6 | fSAMPLING=fDTS/4; N=8 | fSAMPLING=fDTS/8; N=6 | fSAMPLING=fDTS/8; N=8 | fSAMPLING=fDTS/16; N=5 | fSAMPLING=fDTS/16; N=6 | fSAMPLING=fDTS/16; N=8 | fSAMPLING=fDTS/32; N=5 | fSAMPLING=fDTS/32; N=6 | fSAMPLING=fDTS/32; N=8
      mask Callback filterstr: stm32f4_encoderread_callback('filterstr');
      mask Callback sampletimestr: stm32f4_encoderread_callback('sampletimestr');
      mask Callback blockid: stm32f4_encoderread_callback('blockid');
      mask Display: text(0.05, 0.5, 'Timer: 2\nInput pins [CH_A, CH_B]: [A0,A1]\nRST Counter: No\nTs (sec): -1','ver','middle','hor','left');port_label('output', 1, 'Direction');port_label('output', 2, 'Position (count)')
  Obr_sv_left : Subsystem
  Obr_sv_right : Subsystem
  "PS_right " : Subsystem
  ZP_left : Subsystem
  left : Subsystem
  right : Subsystem
  Ps_left : Outport
  wires:
  Encoder Read/1 -> Obr_sv_right/1(In1)
  Encoder Read/2 -> Obr_sv_right/2(In2)
  left/1(Out1) -> Basic PWM1/3
  right/2(Out2) -> Basic PWM1/1
  left/2(Out2) -> Basic PWM1/4
  Obr_sv_left/1(Out1) -> left/2(Obr_sv), Ps_left/1
  Obr_sv_right/1(Out1) -> right/2(Obr_sv)
  right/1(Out1) -> Basic PWM1/2
  Encoder Read1/1 -> Obr_sv_left/1(In1)
  Encoder Read1/2 -> Obr_sv_left/2(In2)
  "PS_right "/1("out1 ") -> right/1(Zadanie)
  Right_cm/1 -> "PS_right "/1(mm)
  Left_cm/1 -> ZP_left/1(mm)
  ZP_left/1("out1 ") -> left/1(Zadanie)

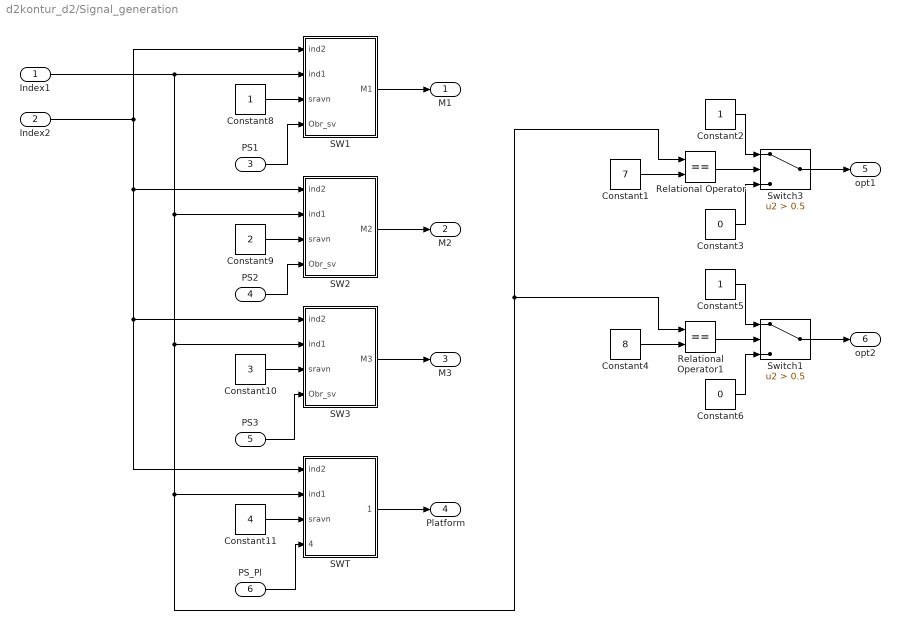
== system d2kontur_d2/Signal_generation ==
  Index1 : Inport
  Index2 : Inport  Port=2
  PS1 : Inport  Port=3
  PS2 : Inport  Port=4
  PS3 : Inport  Port=5
  PS_Pl : Inport  Port=6
  Constant1 : Constant  Value=7
  Constant10 : Constant  Value=3
  Constant11 : Constant  Value=4
  Constant2 : Constant
  Constant3 : Constant  Value=0
  Constant4 : Constant  Value=8
  Constant5 : Constant
  Constant6 : Constant  Value=0
  Constant8 : Constant
  Constant9 : Constant  Value=2
  Relational Operator : RelationalOperator  Operator===  OutDataTypeStr=boolean
  Relational Operator1 : RelationalOperator  Operator===  OutDataTypeStr=boolean
  SW1 : Subsystem
  SW2 : Subsystem
  SW3 : Subsystem
  SWT : Subsystem
  Switch1 : Switch  Criteria=u2 > Threshold  Threshold=0.5
  Switch3 : Switch  Criteria=u2 > Threshold  Threshold=0.5
  M1 : Outport
  M2 : Outport  Port=2
  M3 : Outport  Port=3
  Platform : Outport  Port=4
  opt1 : Outport  Port=5
  opt2 : Outport  Port=6
  wires:
  Constant11/1 -> SWT/3(sravn)
  PS3/1 -> SW3/4("Obr_sv ")
  Constant10/1 -> SW3/3(sravn)
  Constant8/1 -> SW1/3(sravn)
  PS_Pl/1 -> SWT/4("Obr_sv ")
  PS2/1 -> SW2/4("Obr_sv ")
  SW2/1(M2) -> M2/1
  Constant9/1 -> SW2/3(sravn)
  Index2/1 -> SW2/1(ind2), SW3/1(ind2), SWT/1(ind2), SW1/1(ind2)
  SW1/1(M1) -> M1/1
  SW3/1(M3) -> M3/1
  SWT/1(Platform) -> Platform/1
  PS1/1 -> SW1/4("Obr_sv ")
  Constant1/1 -> Relational Operator/2
  Relational Operator/1 -> Switch3/2
  Constant2/1 -> Switch3/1
  Constant3/1 -> Switch3/3
  Switch3/1 -> opt1/1
  Index1/1 -> SW1/2(ind1), SW2/2(ind1), SW3/2(ind1), Relational Operator/1, Relational Operator1/1, SWT/2(ind1)
  Constant4/1 -> Relational Operator1/2
  Relational Operator1/1 -> Switch1/2
  Constant5/1 -> Switch1/1
  Constant6/1 -> Switch1/3
  Switch1/1 -> opt2/1

== system d2kontur_d2/Manipulator/Grab ==
  ind1 : Inport
  Constant14 : Constant  Value=6  OutDataTypeStr=double
  Constant2 : Constant  Value=9  OutDataTypeStr=double
  Constant3 : Constant  OutDataTypeStr=double
  Constant4 : Constant  Value=0  OutDataTypeStr=double
  Discrete-Time Integrator3 : DiscreteIntegrator  gainval=1  ExternalReset=rising  InitialCondition=7  SampleTime=0.001
  Gain5 : Gain  Gain=2
  Relational Operator1 : RelationalOperator  Operator===  OutDataTypeStr=boolean
  Relational Operator2 : RelationalOperator  Operator===  OutDataTypeStr=boolean
  Saturation5 : Saturate  UpperLimit=10  LowerLimit=7
  Switch1 : Switch  Criteria=u2 > Threshold  Threshold=0.5
  pwm : Outport
  wires:
  Gain5/1 -> Discrete-Time Integrator3/1
  Saturation5/1 -> pwm/1
  Discrete-Time Integrator3/1 -> Saturation5/1
  Switch1/1 -> Gain5/1
  Relational Operator1/1 -> Switch1/2
  Constant3/1 -> Switch1/1
  Constant4/1 -> Switch1/3
  ind1/1 -> Relational Operator2/1, Relational Operator1/2
  Constant14/1 -> Relational Operator1/1
  Constant2/1 -> Relational Operator2/2
  Relational Operator2/1 -> Discrete-Time Integrator3/2

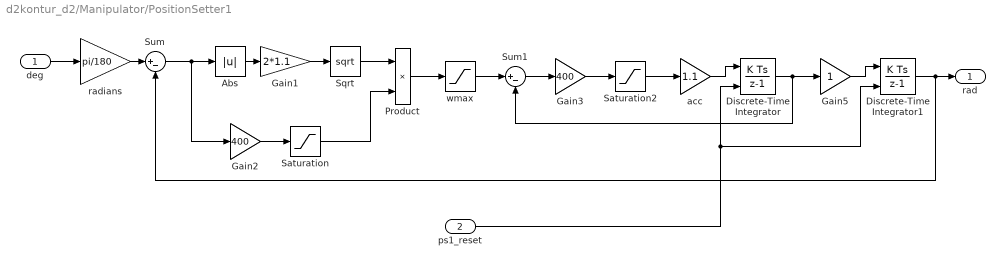
== system d2kontur_d2/Manipulator/PositionSetter1  ==
  "deg " : Inport
  ps1_reset : Inport  Port=2
  Abs : Abs
  Discrete-Time Integrator : DiscreteIntegrator  ExternalReset=rising  SampleTime=0.001
  Discrete-Time Integrator1 : DiscreteIntegrator  ExternalReset=rising  SampleTime=0.001
  Gain1 : Gain  Gain=2*1.1
  Gain2 : Gain  Gain=400
  Gain3 : Gain  Gain=400
  Gain5 : Gain
  Product : Product
  Saturation : Saturate  UpperLimit=1  LowerLimit=-1
  Saturation2 : Saturate  UpperLimit=1  LowerLimit=-1
  Sqrt : Sqrt  SaturateOnIntegerOverflow=on
  Sum : Sum  Inputs=|+-
  Sum1 : Sum  Inputs=|+-
  acc : Gain  Gain=1.1
  radians : Gain  Gain=pi/180
  wmax : Saturate  UpperLimit=0.8  LowerLimit=-0.8
  "rad " : Outport
  wires:
  radians/1 -> Sum/1
  "deg "/1 -> radians/1
  Abs/1 -> Gain1/1
  Sum/1 -> Gain2/1, Abs/1
  Gain1/1 -> Sqrt/1
  Sqrt/1 -> Product/1
  Gain3/1 -> Saturation2/1
  wmax/1 -> Sum1/1
  acc/1 -> Discrete-Time Integrator/1
  Saturation/1 -> Product/2
  Discrete-Time Integrator1/1 -> "rad "/1, Sum/2
  Product/1 -> wmax/1
  Gain5/1 -> Discrete-Time Integrator1/1
  Sum1/1 -> Gain3/1
  Gain2/1 -> Saturation/1
  Discrete-Time Integrator/1 -> Gain5/1, Sum1/2
  Saturation2/1 -> acc/1
  ps1_reset/1 -> Discrete-Time Integrator1/2, Discrete-Time Integrator/2

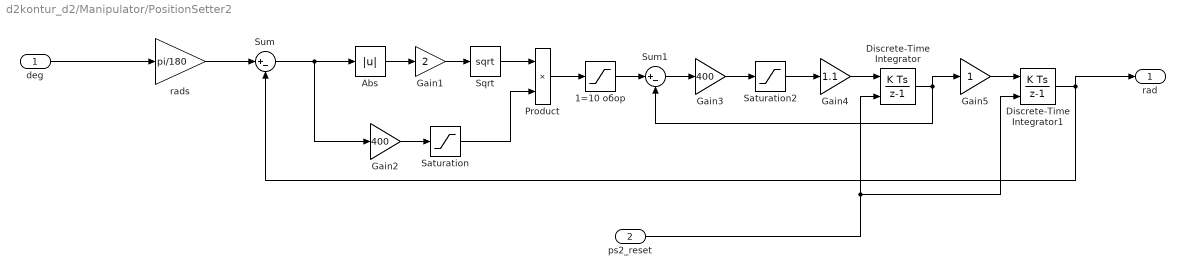
== system d2kontur_d2/Manipulator/PositionSetter2 ==
  deg : Inport
  ps2_reset : Inport  Port=2
  1=10 обор : Saturate  UpperLimit=0.8  LowerLimit=-0.8
  Abs : Abs
  Discrete-Time Integrator : DiscreteIntegrator  ExternalReset=rising  SampleTime=0.001
  Discrete-Time Integrator1 : DiscreteIntegrator  ExternalReset=rising  SampleTime=0.001
  Gain1 : Gain  Gain=2
  Gain2 : Gain  Gain=400
  Gain3 : Gain  Gain=400
  Gain4 : Gain  Gain=1.1
  Gain5 : Gain
  Product : Product
  Saturation : Saturate  UpperLimit=1  LowerLimit=-1
  Saturation2 : Saturate  UpperLimit=1  LowerLimit=-1
  Sqrt : Sqrt  SaturateOnIntegerOverflow=on
  Sum : Sum  Inputs=|+-
  Sum1 : Sum  Inputs=|+-
  rads : Gain  Gain=pi/180
  rad : Outport
  wires:
  rads/1 -> Sum/1
  deg/1 -> rads/1
  Abs/1 -> Gain1/1
  Sum/1 -> Gain2/1, Abs/1
  Gain1/1 -> Sqrt/1
  Sqrt/1 -> Product/1
  Gain3/1 -> Saturation2/1
  1=10 обор/1 -> Sum1/1
  Gain4/1 -> Discrete-Time Integrator/1
  Saturation/1 -> Product/2
  Discrete-Time Integrator1/1 -> rad/1, Sum/2
  Product/1 -> 1=10 обор/1
  Gain5/1 -> Discrete-Time Integrator1/1
  Sum1/1 -> Gain3/1
  Gain2/1 -> Saturation/1
  Discrete-Time Integrator/1 -> Gain5/1, Sum1/2
  Saturation2/1 -> Gain4/1
  ps2_reset/1 -> Discrete-Time Integrator1/2, Discrete-Time Integrator/2

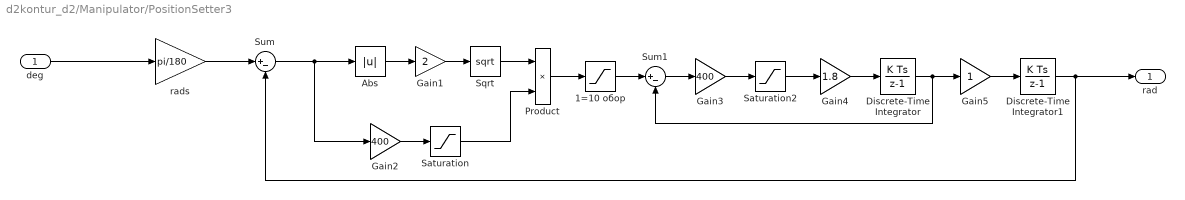
== system d2kontur_d2/Manipulator/PositionSetter3 ==
  deg : Inport
  1=10 обор : Saturate  UpperLimit=2  LowerLimit=-2
  Abs : Abs
  Discrete-Time Integrator : DiscreteIntegrator  SampleTime=0.001
  Discrete-Time Integrator1 : DiscreteIntegrator  SampleTime=0.001
  Gain1 : Gain  Gain=2
  Gain2 : Gain  Gain=400
  Gain3 : Gain  Gain=400
  Gain4 : Gain  Gain=1.8
  Gain5 : Gain
  Product : Product
  Saturation : Saturate  UpperLimit=1  LowerLimit=-1
  Saturation2 : Saturate  UpperLimit=1  LowerLimit=-1
  Sqrt : Sqrt  SaturateOnIntegerOverflow=on
  Sum : Sum  Inputs=|+-
  Sum1 : Sum  Inputs=|+-
  rads : Gain  Gain=pi/180
  rad : Outport
  wires:
  Saturation2/1 -> Gain4/1
  Discrete-Time Integrator/1 -> Sum1/2, Gain5/1
  Gain2/1 -> Saturation/1
  Sum1/1 -> Gain3/1
  Gain5/1 -> Discrete-Time Integrator1/1
  Product/1 -> 1=10 обор/1
  Discrete-Time Integrator1/1 -> Sum/2, rad/1
  Saturation/1 -> Product/2
  Gain4/1 -> Discrete-Time Integrator/1
  1=10 обор/1 -> Sum1/1
  Gain3/1 -> Saturation2/1
  Sqrt/1 -> Product/1
  Gain1/1 -> Sqrt/1
  Sum/1 -> Abs/1, Gain2/1
  Abs/1 -> Gain1/1
  deg/1 -> rads/1
  rads/1 -> Sum/1

== system d2kontur_d2/Manipulator/System1 ==
  PS(1) : Inport
  enc_reset : Inport  Port=2
  Gain1 : Gain  Gain=-1  OutDataTypeStr=double
  Gain4 : Gain  OutDataTypeStr=double
  Mux : Mux  Inputs=2
  PositionFeedback : Subsystem
  Saturation : Saturate  UpperLimit=40  LowerLimit=0  SampleTime=0.001
  Saturation1 : Saturate  UpperLimit=0  LowerLimit=-40  SampleTime=0.001
  Sum : Sum  Inputs=|+-
  k : Gain  Gain=5450
  rad_grad : Gain  Gain=180/pi
  PWM(1) : Outport
  fi1 : Outport  Port=2
  wires:
  Saturation1/1 -> Gain1/1
  Saturation/1 -> Gain4/1
  Sum/1 -> k/1
  PS(1)/1 -> Sum/1
  Gain1/1 -> Mux/1
  Gain4/1 -> Mux/2
  k/1 -> Saturation1/1, Saturation/1
  rad_grad/1 -> fi1/1
  Mux/1 -> PWM(1)/1
  PositionFeedback/1(ps_rad) -> Sum/2, rad_grad/1
  enc_reset/1 -> PositionFeedback/Enable

== system d2kontur_d2/Manipulator/System2 ==
  PS(2) : Inport
  enc2_reset : Inport  Port=2
  " " : Gain  Gain=3650
  Gain1 : Gain  Gain=-1  OutDataTypeStr=double
  Gain4 : Gain  OutDataTypeStr=double
  Mux : Mux  Inputs=2
  Saturation : Saturate  UpperLimit=100  LowerLimit=0  SampleTime=0.001
  Saturation1 : Saturate  UpperLimit=0  LowerLimit=-100  SampleTime=0.001
  Subsystem : Subsystem
  Sum : Sum  Inputs=|+-
  k2 : Gain  Gain=180/pi
  PWM(2) : Outport
  fi2 : Outport  Port=2
  wires:
  Mux/1 -> PWM(2)/1
  Gain4/1 -> Mux/1
  Gain1/1 -> Mux/2
  Saturation1/1 -> Gain1/1
  Saturation/1 -> Gain4/1
  Sum/1 -> " "/1
  PS(2)/1 -> Sum/1
  " "/1 -> Saturation/1, Saturation1/1
  k2/1 -> fi2/1
  Subsystem/1(oc_rad) -> k2/1, Sum/2
  enc2_reset/1 -> Subsystem/Enable
